simulink model "LinearModel"  (R2022b)
settings: Solver=VariableStepAuto  StartTime=0.0  StopTime=10.0  RelTol=1e-3
undefined symbols (not defined in the file): A, B, C, C_pid, Cz_euler, Cz_zoh, D, G
libraries: simulink x1
settings Model: Creator=tumisangramotlhwa  LastModifiedBy=tumisangramotlhwa

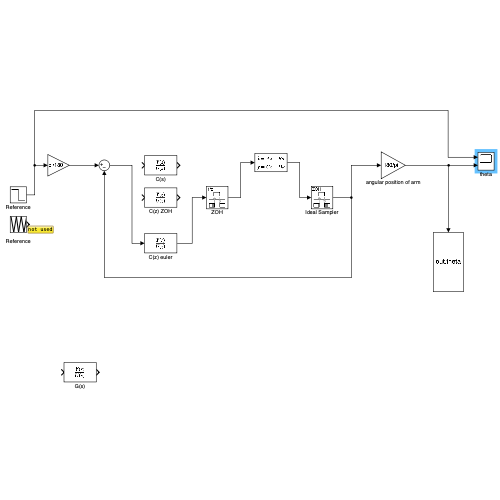
[thumbnail: Simulink's stored preview of the top-level diagram]
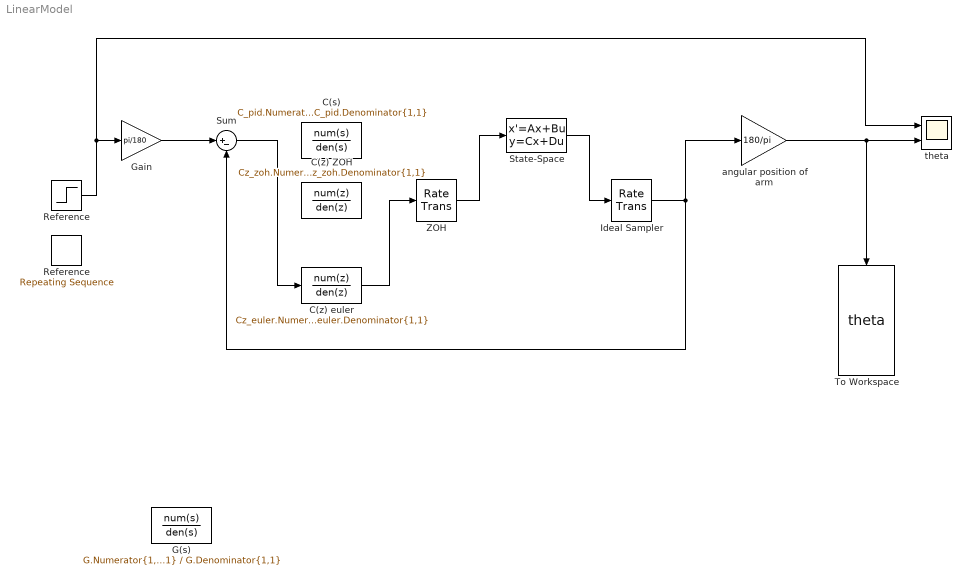
== system LinearModel ==
  " Reference" : simulink/Sources/Repeating Sequence  rep_seq_t=[0 2 4]  rep_seq_y=[45 15 45]
  C(s) : TransferFcn  Numerator=C_pid.Numerator{1,1}  Denominator=C_pid.Denominator{1,1}
  C(z) ZOH : DiscreteTransferFcn  Numerator=Cz_zoh.Numerator{1,1}  Denominator=Cz_zoh.Denominator{1,1}
  C(z) euler : DiscreteTransferFcn  Numerator=Cz_euler.Numerator{1,1}  Denominator=Cz_euler.Denominator{1,1}
  G(s) : TransferFcn  Numerator=G.Numerator{1,1}  Denominator=G.Denominator{1,1}
  Gain : Gain  Gain=pi/180
  Ideal Sampler : RateTransition  OutPortSampleTime=Ts
  Reference : Step  Time=5  Before=45  After=15  SampleTime=0
  State-Space : StateSpace  A=A  B=B  C=C  D=D  InitialCondition=[45*pi/180;45*pi/180;0;0;0]
  Sum : Sum  Inputs=|+-
  To Workspace : ToWorkspace  VariableName=theta  SampleTime=-1
  ZOH : RateTransition
  angular position of arm : Gain  Gain=180/pi
  theta : Scope  NumInputPorts=2
  wires:
  Ideal Sampler/1 -> angular position of arm/1, Sum/2
  C(z) euler/1 -> ZOH/1
  angular position of arm/1 -> theta/2, To Workspace/1
  Gain/1 -> Sum/1
  Sum/1 -> C(z) euler/1
  State-Space/1 -> Ideal Sampler/1
  ZOH/1 -> State-Space/1
  Reference/1 -> Gain/1, theta/1
